simulink model "offboard_SSC_simscape"  (R2025b)
settings: Solver=ode23t  StartTime=0.0  StopTime=0.3  RelTol=1e-3
undefined symbols (not defined in the file): PLL_3ph__class, V_ref
libraries: fl_lib x39, nesl_utility x20, ee_lib x9, simulink x6, eeTransforms x2, batteryecm_lib x1, eeSinusoidalMeasurement x1
(part 2 of 2)

== system offboard_SSC_simscape/Subsystem1 ==
  Va : Inport
  Va1 : Inport  Port=2
  Add1 : Sum
  Constant8 : Constant  Value=0.5
  Divide : Product  Inputs=*/
  Logical Operator1 : Logic  Operator=NOT  AllPortsSameDT=off  OutDataTypeStr=boolean
  Rate Transition : RateTransition  OutPortSampleTime=1e-7
  Rate Transition1 : RateTransition  OutPortSampleTime=1e-7
  Relational Operator : RelationalOperator  OutDataTypeStr=boolean  ZeroCross=off  InputSameDT=off
  Repeating Sequence : simulink/Sources/Repeating Sequence  rep_seq_t=[0 1/30000/2 1/30000]  rep_seq_y=[0 1 0]
  Scope1 : Scope  NumInputPorts=2
      settings: ActiveDisplayYMinimum=-0.12496  ActiveDisplayYMaximum=1.12466  DataLoggingVariableName=ScopeData3
  Scope2 : Scope  NumInputPorts=2
      settings: ActiveDisplayYMinimum=-0.59999  ActiveDisplayYMaximum=3.15933
  Scope3 : Scope  NumInputPorts=2
      settings: ActiveDisplayYMinimum=-0.125  ActiveDisplayYMaximum=1.125  DataLoggingVariableName=ScopeData2
  Vcomp*2 : Constant  Value=1200
  A : Outport
  A' : Outport  Port=2
  wires:
  Va/1 -> Rate Transition/1
  Divide/1 -> Add1/1
  Add1/1 -> Scope2/1, Relational Operator/2
  Constant8/1 -> Add1/2
  Repeating Sequence/1 -> Scope1/1, Relational Operator/1
  Logical Operator1/1 -> Scope3/1, A/1
  Relational Operator/1 -> Scope3/2, A'/1, Logical Operator1/1
  Va1/1 -> Rate Transition1/1
  Rate Transition/1 -> Divide/1
  Rate Transition1/1 -> Divide/2

== system offboard_SSC_simscape/Subsystem2 ==
  Vb : Inport
  Va : Inport  Port=2
  Add1 : Sum
  Constant8 : Constant  Value=0.5
  Divide : Product  Inputs=*/
  Logical Operator1 : Logic  Operator=NOT  AllPortsSameDT=off  OutDataTypeStr=boolean
  Rate Transition : RateTransition  OutPortSampleTime=1e-7
  Rate Transition1 : RateTransition  OutPortSampleTime=1e-7
  Relational Operator : RelationalOperator  OutDataTypeStr=boolean  ZeroCross=off  InputSameDT=off
  Repeating Sequence : simulink/Sources/Repeating Sequence  rep_seq_t=[0 1/30000/2 1/30000]  rep_seq_y=[0 1 0]
  Scope1 : Scope  NumInputPorts=2
      settings: ActiveDisplayYMinimum=-0.125  ActiveDisplayYMaximum=1.125  DataLoggingVariableName=ScopeData3
  Scope4 : Scope  NumInputPorts=2
      settings: ActiveDisplayYMinimum=-500  ActiveDisplayYMaximum=500  DataLoggingVariableName=ScopeData3
  Vcomp*2 : Constant  Value=1200
  B : Outport
  B' : Outport  Port=2
  wires:
  Vb/1 -> Rate Transition/1
  Divide/1 -> Add1/1
  Add1/1 -> Relational Operator/2, Scope4/2
  Constant8/1 -> Add1/2
  Repeating Sequence/1 -> Scope1/1, Relational Operator/1
  Logical Operator1/1 -> B/1
  Relational Operator/1 -> B'/1, Logical Operator1/1
  Va/1 -> Rate Transition1/1
  Rate Transition/1 -> Divide/1
  Rate Transition1/1 -> Divide/2

== system offboard_SSC_simscape/Subsystem3 ==
  Va : Inport
  Add1 : Sum
  Constant8 : Constant  Value=0.5
  Divide : Product  Inputs=*/
  Logical Operator1 : Logic  Operator=NOT  AllPortsSameDT=off  OutDataTypeStr=boolean
  Rate Transition : RateTransition  OutPortSampleTime=1e-7
  Relational Operator : RelationalOperator  OutDataTypeStr=boolean  ZeroCross=off  InputSameDT=off
  Repeating Sequence : simulink/Sources/Repeating Sequence  rep_seq_t=[0 1/100000/2 1/100000]  rep_seq_y=[0 1 0]
  Scope1 : Scope  NumInputPorts=2
      settings: ActiveDisplayYMinimum=-0.12496  ActiveDisplayYMaximum=1.12466  DataLoggingVariableName=ScopeData3
  Scope2 : Scope  NumInputPorts=2
      settings: ActiveDisplayYMinimum=-0.59999  ActiveDisplayYMaximum=3.15933
  Scope3 : Scope  NumInputPorts=2
      settings: ActiveDisplayYMinimum=-0.125  ActiveDisplayYMaximum=1.125  DataLoggingVariableName=ScopeData2
  Vcomp*2 : Constant  Value=800
  A : Outport
  A' : Outport  Port=2
  wires:
  Va/1 -> Rate Transition/1
  Divide/1 -> Add1/1
  Add1/1 -> Scope2/1, Relational Operator/2
  Constant8/1 -> Add1/2
  Repeating Sequence/1 -> Scope1/1, Relational Operator/1
  Logical Operator1/1 -> Scope3/1, A/1
  Relational Operator/1 -> Scope3/2, A'/1, Logical Operator1/1
  Vcomp*2/1 -> Divide/2
  Rate Transition/1 -> Divide/1

== system offboard_SSC_simscape/Subsystem4 ==
  Vc : Inport
  Va : Inport  Port=2
  Add1 : Sum
  Constant8 : Constant  Value=0.5
  Divide : Product  Inputs=*/
  Logical Operator1 : Logic  Operator=NOT  AllPortsSameDT=off  OutDataTypeStr=boolean
  Rate Transition : RateTransition  OutPortSampleTime=1e-7
  Rate Transition1 : RateTransition  OutPortSampleTime=1e-7
  Relational Operator : RelationalOperator  OutDataTypeStr=boolean  ZeroCross=off  InputSameDT=off
  Repeating Sequence : simulink/Sources/Repeating Sequence  rep_seq_t=[0 1/30000/2 1/30000]  rep_seq_y=[0 1 0]
  Scope1 : Scope  NumInputPorts=2
      settings: ActiveDisplayYMinimum=-0.125  ActiveDisplayYMaximum=1.125  DataLoggingVariableName=ScopeData3
  Scope4 : Scope  NumInputPorts=2
      settings: ActiveDisplayYMinimum=-500  ActiveDisplayYMaximum=500  DataLoggingVariableName=ScopeData3
  Vcomp*2 : Constant  Value=1200
  C : Outport
  C' : Outport  Port=2
  wires:
  Vc/1 -> Rate Transition/1
  Divide/1 -> Add1/1
  Add1/1 -> Relational Operator/2, Scope4/2
  Constant8/1 -> Add1/2
  Repeating Sequence/1 -> Scope1/1, Relational Operator/1
  Logical Operator1/1 -> C/1
  Relational Operator/1 -> C'/1, Logical Operator1/1
  Va/1 -> Rate Transition1/1
  Rate Transition/1 -> Divide/1
  Rate Transition1/1 -> Divide/2

== system offboard_SSC_simscape/Subsystem5 ==
  Va : Inport
  Add1 : Sum
  Constant8 : Constant  Value=0.5
  Divide : Product  Inputs=*/
  Logical Operator1 : Logic  Operator=NOT  AllPortsSameDT=off  OutDataTypeStr=boolean
  Rate Transition : RateTransition  OutPortSampleTime=1e-7
  Relational Operator : RelationalOperator  OutDataTypeStr=boolean  ZeroCross=off  InputSameDT=off
  Repeating Sequence : simulink/Sources/Repeating Sequence  rep_seq_t=[0 1/100000/2 1/100000]  rep_seq_y=[0 1 0]
  Scope1 : Scope  NumInputPorts=2
      settings: ActiveDisplayYMinimum=-0.12496  ActiveDisplayYMaximum=1.12466  DataLoggingVariableName=ScopeData3
  Scope2 : Scope  NumInputPorts=2
      settings: ActiveDisplayYMinimum=-0.59999  ActiveDisplayYMaximum=3.15933
  Scope3 : Scope  NumInputPorts=2
      settings: ActiveDisplayYMinimum=-0.125  ActiveDisplayYMaximum=1.125  DataLoggingVariableName=ScopeData2
  Vcomp*2 : Constant  Value=800
  A : Outport
  A' : Outport  Port=2
  wires:
  Va/1 -> Rate Transition/1
  Divide/1 -> Add1/1
  Add1/1 -> Scope2/1, Relational Operator/2
  Constant8/1 -> Add1/2
  Repeating Sequence/1 -> Scope1/1, Relational Operator/1
  Logical Operator1/1 -> Scope3/1, A/1
  Relational Operator/1 -> Scope3/2, A'/1, Logical Operator1/1
  Vcomp*2/1 -> Divide/2
  Rate Transition/1 -> Divide/1

== system offboard_SSC_simscape/Subsystem6 ==
  Va : Inport
  Add1 : Sum
  Constant8 : Constant  Value=0.5
  Divide : Product  Inputs=*/
  Logical Operator1 : Logic  Operator=NOT  AllPortsSameDT=off  OutDataTypeStr=boolean
  Rate Transition : RateTransition  OutPortSampleTime=1e-7
  Relational Operator : RelationalOperator  OutDataTypeStr=boolean  ZeroCross=off  InputSameDT=off
  Repeating Sequence : simulink/Sources/Repeating Sequence  rep_seq_t=[0 1/100000/2 1/100000]  rep_seq_y=[0 1 0]
  Scope1 : Scope  NumInputPorts=2
      settings: ActiveDisplayYMinimum=-0.12496  ActiveDisplayYMaximum=1.12466  DataLoggingVariableName=ScopeData3
  Scope2 : Scope  NumInputPorts=2
      settings: ActiveDisplayYMinimum=-0.59999  ActiveDisplayYMaximum=3.15933
  Scope3 : Scope  NumInputPorts=2
      settings: ActiveDisplayYMinimum=-0.125  ActiveDisplayYMaximum=1.125  DataLoggingVariableName=ScopeData2
  Vcomp*2 : Constant  Value=800
  A : Outport
  A' : Outport  Port=2
  wires:
  Va/1 -> Rate Transition/1
  Divide/1 -> Add1/1
  Add1/1 -> Scope2/1, Relational Operator/2
  Constant8/1 -> Add1/2
  Repeating Sequence/1 -> Scope1/1, Relational Operator/1
  Logical Operator1/1 -> Scope3/1, A/1
  Relational Operator/1 -> Scope3/2, A'/1, Logical Operator1/1
  Vcomp*2/1 -> Divide/2
  Rate Transition/1 -> Divide/1

== system offboard_SSC_simscape/DC//DC1/S1 ==
  g : Inport
  Diode : fl_lib/Electrical/Electrical Elements/Diode  Vf=1e-3 V  Ron=1e-2 Ohm  Goff=1e-5 1/Ohm  i_specify=off  i_priority=None  i=0 A  i_nominal_specify=off  i_nominal_value=1  i_nominal_unit=A  v_specify=off  v_priority=None  v=0 V  v_nominal_specify=off  v_nominal_value=1  v_nominal_unit=V
  S1 : fl_lib/Electrical/Electrical Elements/Switch  R_closed=0.1 Ohm  G_open=1e-5 1/Ohm  Threshold=0.5  i_specify=off  i_priority=None  i=0 A  i_nominal_specify=off  i_nominal_value=1  i_nominal_unit=A  v_specify=off  v_priority=None  v=0 V  v_nominal_specify=off  v_nominal_value=1  v_nominal_unit=V
  Simulink-PS Converter : nesl_utility/Simulink-PS Converter  PhysicalDomain=network_engine_domain  SubClassName=ps_input  LeftPortType=input  RightPortType=output  PseudoPeriodic=off  Frequencies=[]  NoiseDistribution=none  NoiseParameters=[]  Unit=1  AffineConversion=off  FilteringAndDerivatives=zero  SimscapeFilterOrder=1  InputFilterTimeConstant=0.001  UdotUserProvided=0
  + : PMIOPort  Side=Left
  - : PMIOPort  Port=2  Side=Right
  wires:
  g/1 -> Simulink-PS Converter/1
  connections:
  S1/RConn2 -- -/RConn1 -- Diode/LConn1
  Diode/RConn1 -- +/RConn1 -- S1/LConn1
  Simulink-PS Converter/RConn1 -- S1/RConn1

== system offboard_SSC_simscape/DC//DC1/S2 ==
  g : Inport
  Diode : fl_lib/Electrical/Electrical Elements/Diode  Vf=1e-3 V  Ron=1e-2 Ohm  Goff=1e-5 1/Ohm  i_specify=off  i_priority=None  i=0 A  i_nominal_specify=off  i_nominal_value=1  i_nominal_unit=A  v_specify=off  v_priority=None  v=0 V  v_nominal_specify=off  v_nominal_value=1  v_nominal_unit=V
  S1 : fl_lib/Electrical/Electrical Elements/Switch  R_closed=0.1 Ohm  G_open=1e-5 1/Ohm  Threshold=0.5  i_specify=off  i_priority=None  i=0 A  i_nominal_specify=off  i_nominal_value=1  i_nominal_unit=A  v_specify=off  v_priority=None  v=0 V  v_nominal_specify=off  v_nominal_value=1  v_nominal_unit=V
  Simulink-PS Converter : nesl_utility/Simulink-PS Converter  PhysicalDomain=network_engine_domain  SubClassName=ps_input  LeftPortType=input  RightPortType=output  PseudoPeriodic=off  Frequencies=[]  NoiseDistribution=none  NoiseParameters=[]  Unit=1  AffineConversion=off  FilteringAndDerivatives=zero  SimscapeFilterOrder=1  InputFilterTimeConstant=0.001  UdotUserProvided=0
  + : PMIOPort  Side=Left
  - : PMIOPort  Port=2  Side=Right
  wires:
  g/1 -> Simulink-PS Converter/1
  connections:
  Simulink-PS Converter/RConn1 -- S1/RConn1
  S1/LConn1 -- +/RConn1 -- Diode/RConn1
  Diode/LConn1 -- -/RConn1 -- S1/RConn2

== system offboard_SSC_simscape/DC//DC2/S1 ==
  g : Inport
  Diode : fl_lib/Electrical/Electrical Elements/Diode  Vf=1e-3 V  Ron=1e-2 Ohm  Goff=1e-5 1/Ohm  i_specify=off  i_priority=None  i=0 A  i_nominal_specify=off  i_nominal_value=1  i_nominal_unit=A  v_specify=off  v_priority=None  v=0 V  v_nominal_specify=off  v_nominal_value=1  v_nominal_unit=V
  S1 : fl_lib/Electrical/Electrical Elements/Switch  R_closed=0.1 Ohm  G_open=1e-5 1/Ohm  Threshold=0.5  i_specify=off  i_priority=None  i=0 A  i_nominal_specify=off  i_nominal_value=1  i_nominal_unit=A  v_specify=off  v_priority=None  v=0 V  v_nominal_specify=off  v_nominal_value=1  v_nominal_unit=V
  Simulink-PS Converter : nesl_utility/Simulink-PS Converter  PhysicalDomain=network_engine_domain  SubClassName=ps_input  LeftPortType=input  RightPortType=output  PseudoPeriodic=off  Frequencies=[]  NoiseDistribution=none  NoiseParameters=[]  Unit=1  AffineConversion=off  FilteringAndDerivatives=zero  SimscapeFilterOrder=1  InputFilterTimeConstant=0.001  UdotUserProvided=0
  + : PMIOPort  Side=Left
  - : PMIOPort  Port=2  Side=Right
  wires:
  g/1 -> Simulink-PS Converter/1
  connections:
  S1/RConn2 -- -/RConn1 -- Diode/LConn1
  Diode/RConn1 -- +/RConn1 -- S1/LConn1
  Simulink-PS Converter/RConn1 -- S1/RConn1

== system offboard_SSC_simscape/DC//DC2/S2 ==
  g : Inport
  Diode : fl_lib/Electrical/Electrical Elements/Diode  Vf=1e-3 V  Ron=1e-2 Ohm  Goff=1e-5 1/Ohm  i_specify=off  i_priority=None  i=0 A  i_nominal_specify=off  i_nominal_value=1  i_nominal_unit=A  v_specify=off  v_priority=None  v=0 V  v_nominal_specify=off  v_nominal_value=1  v_nominal_unit=V
  S1 : fl_lib/Electrical/Electrical Elements/Switch  R_closed=0.1 Ohm  G_open=1e-5 1/Ohm  Threshold=0.5  i_specify=off  i_priority=None  i=0 A  i_nominal_specify=off  i_nominal_value=1  i_nominal_unit=A  v_specify=off  v_priority=None  v=0 V  v_nominal_specify=off  v_nominal_value=1  v_nominal_unit=V
  Simulink-PS Converter : nesl_utility/Simulink-PS Converter  PhysicalDomain=network_engine_domain  SubClassName=ps_input  LeftPortType=input  RightPortType=output  PseudoPeriodic=off  Frequencies=[]  NoiseDistribution=none  NoiseParameters=[]  Unit=1  AffineConversion=off  FilteringAndDerivatives=zero  SimscapeFilterOrder=1  InputFilterTimeConstant=0.001  UdotUserProvided=0
  + : PMIOPort  Side=Left
  - : PMIOPort  Port=2  Side=Right
  wires:
  g/1 -> Simulink-PS Converter/1
  connections:
  Simulink-PS Converter/RConn1 -- S1/RConn1
  S1/LConn1 -- +/RConn1 -- Diode/RConn1
  Diode/LConn1 -- -/RConn1 -- S1/RConn2

== system offboard_SSC_simscape/DC//DC3/S1 ==
  g : Inport
  Diode : fl_lib/Electrical/Electrical Elements/Diode  Vf=1e-3 V  Ron=1e-2 Ohm  Goff=1e-5 1/Ohm  i_specify=off  i_priority=None  i=0 A  i_nominal_specify=off  i_nominal_value=1  i_nominal_unit=A  v_specify=off  v_priority=None  v=0 V  v_nominal_specify=off  v_nominal_value=1  v_nominal_unit=V
  S1 : fl_lib/Electrical/Electrical Elements/Switch  R_closed=0.1 Ohm  G_open=1e-5 1/Ohm  Threshold=0.5  i_specify=off  i_priority=None  i=0 A  i_nominal_specify=off  i_nominal_value=1  i_nominal_unit=A  v_specify=off  v_priority=None  v=0 V  v_nominal_specify=off  v_nominal_value=1  v_nominal_unit=V
  Simulink-PS Converter : nesl_utility/Simulink-PS Converter  PhysicalDomain=network_engine_domain  SubClassName=ps_input  LeftPortType=input  RightPortType=output  PseudoPeriodic=off  Frequencies=[]  NoiseDistribution=none  NoiseParameters=[]  Unit=1  AffineConversion=off  FilteringAndDerivatives=zero  SimscapeFilterOrder=1  InputFilterTimeConstant=0.001  UdotUserProvided=0
  + : PMIOPort  Side=Left
  - : PMIOPort  Port=2  Side=Right
  wires:
  g/1 -> Simulink-PS Converter/1
  connections:
  S1/RConn2 -- -/RConn1 -- Diode/LConn1
  Diode/RConn1 -- +/RConn1 -- S1/LConn1
  Simulink-PS Converter/RConn1 -- S1/RConn1

== system offboard_SSC_simscape/DC//DC3/S2 ==
  g : Inport
  Diode : fl_lib/Electrical/Electrical Elements/Diode  Vf=1e-3 V  Ron=1e-2 Ohm  Goff=1e-5 1/Ohm  i_specify=off  i_priority=None  i=0 A  i_nominal_specify=off  i_nominal_value=1  i_nominal_unit=A  v_specify=off  v_priority=None  v=0 V  v_nominal_specify=off  v_nominal_value=1  v_nominal_unit=V
  S1 : fl_lib/Electrical/Electrical Elements/Switch  R_closed=0.1 Ohm  G_open=1e-5 1/Ohm  Threshold=0.5  i_specify=off  i_priority=None  i=0 A  i_nominal_specify=off  i_nominal_value=1  i_nominal_unit=A  v_specify=off  v_priority=None  v=0 V  v_nominal_specify=off  v_nominal_value=1  v_nominal_unit=V
  Simulink-PS Converter : nesl_utility/Simulink-PS Converter  PhysicalDomain=network_engine_domain  SubClassName=ps_input  LeftPortType=input  RightPortType=output  PseudoPeriodic=off  Frequencies=[]  NoiseDistribution=none  NoiseParameters=[]  Unit=1  AffineConversion=off  FilteringAndDerivatives=zero  SimscapeFilterOrder=1  InputFilterTimeConstant=0.001  UdotUserProvided=0
  + : PMIOPort  Side=Left
  - : PMIOPort  Port=2  Side=Right
  wires:
  g/1 -> Simulink-PS Converter/1
  connections:
  Simulink-PS Converter/RConn1 -- S1/RConn1
  S1/LConn1 -- +/RConn1 -- Diode/RConn1
  Diode/LConn1 -- -/RConn1 -- S1/RConn2

== system offboard_SSC_simscape/Front End/S1 ==
  g : Inport
  Diode : fl_lib/Electrical/Electrical Elements/Diode  Vf=1e-3 V  Ron=1e-2 Ohm  Goff=1e-5 1/Ohm  i_specify=off  i_priority=None  i=0 A  i_nominal_specify=off  i_nominal_value=1  i_nominal_unit=A  v_specify=off  v_priority=None  v=0 V  v_nominal_specify=off  v_nominal_value=1  v_nominal_unit=V
  S1 : fl_lib/Electrical/Electrical Elements/Switch  R_closed=0.1 Ohm  G_open=1e-5 1/Ohm  Threshold=0.5  i_specify=off  i_priority=None  i=0 A  i_nominal_specify=off  i_nominal_value=1  i_nominal_unit=A  v_specify=off  v_priority=None  v=0 V  v_nominal_specify=off  v_nominal_value=1  v_nominal_unit=V
  Simulink-PS Converter : nesl_utility/Simulink-PS Converter  PhysicalDomain=network_engine_domain  SubClassName=ps_input  LeftPortType=input  RightPortType=output  PseudoPeriodic=off  Frequencies=[]  NoiseDistribution=none  NoiseParameters=[]  Unit=1  AffineConversion=off  FilteringAndDerivatives=zero  SimscapeFilterOrder=1  InputFilterTimeConstant=0.001  UdotUserProvided=0
  + : PMIOPort  Side=Left
  - : PMIOPort  Port=2  Side=Right
  wires:
  g/1 -> Simulink-PS Converter/1
  connections:
  S1/RConn2 -- -/RConn1 -- Diode/LConn1
  Diode/RConn1 -- S1/LConn1 -- +/RConn1
  Simulink-PS Converter/RConn1 -- S1/RConn1

== system offboard_SSC_simscape/Front End/S2 ==
  g : Inport
  Diode : fl_lib/Electrical/Electrical Elements/Diode  Vf=1e-3 V  Ron=1e-2 Ohm  Goff=1e-5 1/Ohm  i_specify=off  i_priority=None  i=0 A  i_nominal_specify=off  i_nominal_value=1  i_nominal_unit=A  v_specify=off  v_priority=None  v=0 V  v_nominal_specify=off  v_nominal_value=1  v_nominal_unit=V
  S1 : fl_lib/Electrical/Electrical Elements/Switch  R_closed=0.1 Ohm  G_open=1e-5 1/Ohm  Threshold=0.5  i_specify=off  i_priority=None  i=0 A  i_nominal_specify=off  i_nominal_value=1  i_nominal_unit=A  v_specify=off  v_priority=None  v=0 V  v_nominal_specify=off  v_nominal_value=1  v_nominal_unit=V
  Simulink-PS Converter : nesl_utility/Simulink-PS Converter  PhysicalDomain=network_engine_domain  SubClassName=ps_input  LeftPortType=input  RightPortType=output  PseudoPeriodic=off  Frequencies=[]  NoiseDistribution=none  NoiseParameters=[]  Unit=1  AffineConversion=off  FilteringAndDerivatives=zero  SimscapeFilterOrder=1  InputFilterTimeConstant=0.001  UdotUserProvided=0
  + : PMIOPort  Side=Left
  - : PMIOPort  Port=2  Side=Right
  wires:
  g/1 -> Simulink-PS Converter/1
  connections:
  Simulink-PS Converter/RConn1 -- S1/RConn1
  S1/LConn1 -- +/RConn1 -- Diode/RConn1
  Diode/LConn1 -- S1/RConn2 -- -/RConn1

== system offboard_SSC_simscape/Front End/S3 ==
  g : Inport
  Diode : fl_lib/Electrical/Electrical Elements/Diode  Vf=1e-3 V  Ron=1e-2 Ohm  Goff=1e-5 1/Ohm  i_specify=off  i_priority=None  i=0 A  i_nominal_specify=off  i_nominal_value=1  i_nominal_unit=A  v_specify=off  v_priority=None  v=0 V  v_nominal_specify=off  v_nominal_value=1  v_nominal_unit=V
  S1 : fl_lib/Electrical/Electrical Elements/Switch  R_closed=0.1 Ohm  G_open=1e-5 1/Ohm  Threshold=0.5  i_specify=off  i_priority=None  i=0 A  i_nominal_specify=off  i_nominal_value=1  i_nominal_unit=A  v_specify=off  v_priority=None  v=0 V  v_nominal_specify=off  v_nominal_value=1  v_nominal_unit=V
  Simulink-PS Converter : nesl_utility/Simulink-PS Converter  PhysicalDomain=network_engine_domain  SubClassName=ps_input  LeftPortType=input  RightPortType=output  PseudoPeriodic=off  Frequencies=[]  NoiseDistribution=none  NoiseParameters=[]  Unit=1  AffineConversion=off  FilteringAndDerivatives=zero  SimscapeFilterOrder=1  InputFilterTimeConstant=0.001  UdotUserProvided=0
  + : PMIOPort  Side=Left
  - : PMIOPort  Port=2  Side=Right
  wires:
  g/1 -> Simulink-PS Converter/1
  connections:
  -/RConn1 -- S1/RConn2 -- Diode/LConn1
  Diode/RConn1 -- +/RConn1 -- S1/LConn1
  Simulink-PS Converter/RConn1 -- S1/RConn1

== system offboard_SSC_simscape/Front End/S4 ==
  g : Inport
  Diode : fl_lib/Electrical/Electrical Elements/Diode  Vf=1e-3 V  Ron=1e-2 Ohm  Goff=1e-5 1/Ohm  i_specify=off  i_priority=None  i=0 A  i_nominal_specify=off  i_nominal_value=1  i_nominal_unit=A  v_specify=off  v_priority=None  v=0 V  v_nominal_specify=off  v_nominal_value=1  v_nominal_unit=V
  S1 : fl_lib/Electrical/Electrical Elements/Switch  R_closed=0.1 Ohm  G_open=1e-5 1/Ohm  Threshold=0.5  i_specify=off  i_priority=None  i=0 A  i_nominal_specify=off  i_nominal_value=1  i_nominal_unit=A  v_specify=off  v_priority=None  v=0 V  v_nominal_specify=off  v_nominal_value=1  v_nominal_unit=V
  Simulink-PS Converter : nesl_utility/Simulink-PS Converter  PhysicalDomain=network_engine_domain  SubClassName=ps_input  LeftPortType=input  RightPortType=output  PseudoPeriodic=off  Frequencies=[]  NoiseDistribution=none  NoiseParameters=[]  Unit=1  AffineConversion=off  FilteringAndDerivatives=zero  SimscapeFilterOrder=1  InputFilterTimeConstant=0.001  UdotUserProvided=0
  + : PMIOPort  Side=Left
  - : PMIOPort  Port=2  Side=Right
  wires:
  g/1 -> Simulink-PS Converter/1
  connections:
  Simulink-PS Converter/RConn1 -- S1/RConn1
  S1/LConn1 -- +/RConn1 -- Diode/RConn1
  Diode/LConn1 -- S1/RConn2 -- -/RConn1

== system offboard_SSC_simscape/Front End/S5 ==
  g : Inport
  Diode : fl_lib/Electrical/Electrical Elements/Diode  Vf=1e-3 V  Ron=1e-2 Ohm  Goff=1e-5 1/Ohm  i_specify=off  i_priority=None  i=0 A  i_nominal_specify=off  i_nominal_value=1  i_nominal_unit=A  v_specify=off  v_priority=None  v=0 V  v_nominal_specify=off  v_nominal_value=1  v_nominal_unit=V
  S1 : fl_lib/Electrical/Electrical Elements/Switch  R_closed=0.1 Ohm  G_open=1e-5 1/Ohm  Threshold=0.5  i_specify=off  i_priority=None  i=0 A  i_nominal_specify=off  i_nominal_value=1  i_nominal_unit=A  v_specify=off  v_priority=None  v=0 V  v_nominal_specify=off  v_nominal_value=1  v_nominal_unit=V
  Simulink-PS Converter : nesl_utility/Simulink-PS Converter  PhysicalDomain=network_engine_domain  SubClassName=ps_input  LeftPortType=input  RightPortType=output  PseudoPeriodic=off  Frequencies=[]  NoiseDistribution=none  NoiseParameters=[]  Unit=1  AffineConversion=off  FilteringAndDerivatives=zero  SimscapeFilterOrder=1  InputFilterTimeConstant=0.001  UdotUserProvided=0
  + : PMIOPort  Side=Left
  - : PMIOPort  Port=2  Side=Right
  wires:
  g/1 -> Simulink-PS Converter/1
  connections:
  -/RConn1 -- S1/RConn2 -- Diode/LConn1
  Diode/RConn1 -- +/RConn1 -- S1/LConn1
  Simulink-PS Converter/RConn1 -- S1/RConn1

== system offboard_SSC_simscape/Front End/S6 ==
  g : Inport
  Diode : fl_lib/Electrical/Electrical Elements/Diode  Vf=1e-3 V  Ron=1e-2 Ohm  Goff=1e-5 1/Ohm  i_specify=off  i_priority=None  i=0 A  i_nominal_specify=off  i_nominal_value=1  i_nominal_unit=A  v_specify=off  v_priority=None  v=0 V  v_nominal_specify=off  v_nominal_value=1  v_nominal_unit=V
  S1 : fl_lib/Electrical/Electrical Elements/Switch  R_closed=0.1 Ohm  G_open=1e-5 1/Ohm  Threshold=0.5  i_specify=off  i_priority=None  i=0 A  i_nominal_specify=off  i_nominal_value=1  i_nominal_unit=A  v_specify=off  v_priority=None  v=0 V  v_nominal_specify=off  v_nominal_value=1  v_nominal_unit=V
  Simulink-PS Converter : nesl_utility/Simulink-PS Converter  PhysicalDomain=network_engine_domain  SubClassName=ps_input  LeftPortType=input  RightPortType=output  PseudoPeriodic=off  Frequencies=[]  NoiseDistribution=none  NoiseParameters=[]  Unit=1  AffineConversion=off  FilteringAndDerivatives=zero  SimscapeFilterOrder=1  InputFilterTimeConstant=0.001  UdotUserProvided=0
  + : PMIOPort  Side=Left
  - : PMIOPort  Port=2  Side=Right
  wires:
  g/1 -> Simulink-PS Converter/1
  connections:
  Simulink-PS Converter/RConn1 -- S1/RConn1
  S1/LConn1 -- +/RConn1 -- Diode/RConn1
  Diode/LConn1 -- S1/RConn2 -- -/RConn1
